simulink model "ad_estimator"  (Simulink 9.3)
settings: Solver=VariableStepAuto  StartTime=0.0  StopTime=10000  MaxStep=0.1  RelTol=1e-3
undefined symbols (not defined in the file or in its folder): a1, a2, b, gam, la
settings Model: Creator=jkord  LastModifiedBy=jkord
settings DataIOCC: SaveFormat=Dataset  SignalLoggingSaveFormat=Dataset  ReturnWorkspaceOutputs=on
settings OptimizationCC: LifeSpan=auto
settings DebuggingCC: UnderspecifiedInitializationDetection=Simplified  MergeDetectMultiDrivingBlocksExec=error  FcnCallInpInsideContextMsg=error  SFUnexpectedBacktrackingDiag=error  SFNoUnconditionalDefaultTransitionDiag=error  SFExecutionAtInitializationDiag=warning  ArithmeticOperatorsInVariantConditions=error
settings HardwareCC: ProdBitPerPointer=64  ProdBitPerSizeT=64  ProdBitPerPtrDiffT=64  ProdLargestAtomicFloat=Float  ProdIntDivRoundTo=Zero  ProdEndianess=LittleEndian  ProdWordSize=64  ProdHWDeviceType=Intel->x86-64 (Windows64)
settings ModelReferenceCC: PropagateSignalLabelsOutOfModel=on
settings SFSimCC: SimUseLocalCustomCode=on
settings RTWCC: RTWUseLocalCustomCode=on
settings CodeAppCC: StateflowObjectComments=off
settings GRTTargetCC: TargetLangStandard=C99 (ISO)  CombineOutputUpdateFcns=on  GRTInterface=off
settings ConfigComp: CovMetricSettings=dwe  CovHtmlReporting=off  CovSaveCumulativeToWorkspaceVar=off  CovSaveSingleToWorkspaceVar=off  CovExternalEMLEnable=on

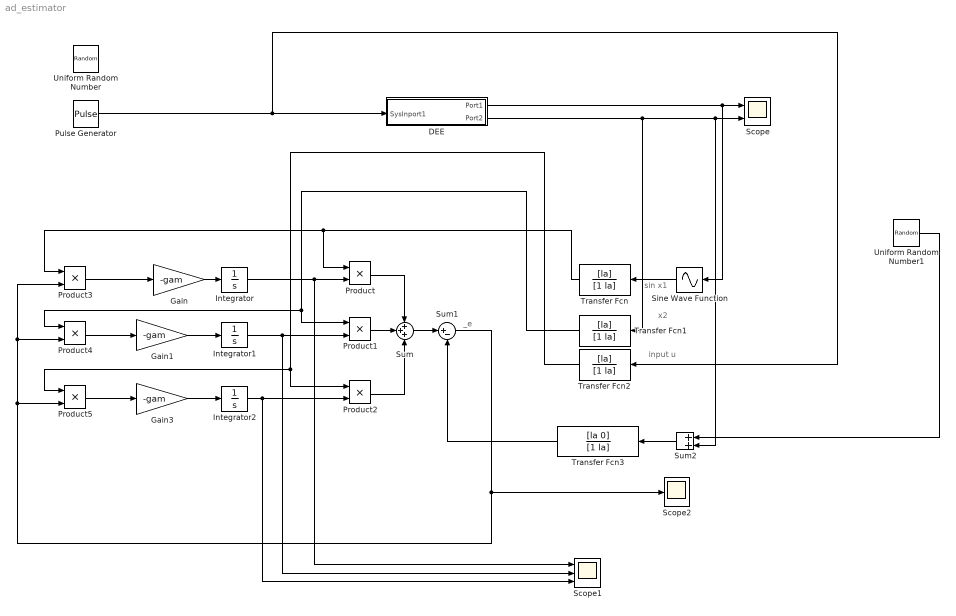
== system ad_estimator ==
  note: _e
  note: input u
  note: x2
  note: sin x1
  DEE : Subsystem  mask(Differential Equation Editor (DEE)){}
      settings: OpenFcn=diffeqed
      mask Display: disp('Differential Equation\n Editor')
  Gain : Gain  Gain=-gam
  Gain1 : Gain  Gain=-gam
  Gain3 : Gain  Gain=-gam
  Integrator : Integrator
  Integrator1 : Integrator
  Integrator2 : Integrator
  Product{,1..5} (6 alike) : Product
  Pulse Generator : DiscretePulseGenerator  PulseType=Time based  Amplitude=0.2  Period=50  PulseWidth=50
  Scope : Scope  NumInputPorts=2
  Scope1 : Scope  NumInputPorts=3
  Scope2 : Scope
  Sine Wave Function : Sin  TimeSource=Use external signal  SampleTime=0
  Sum : Sum  Inputs=+++
  Sum1 : Sum  Inputs=|+-
  Sum2 : Sum
  Transfer Fcn : TransferFcn  Numerator=[la]  Denominator=[1 la]
  Transfer Fcn1 : TransferFcn  Numerator=[la]  Denominator=[1 la]
  Transfer Fcn2 : TransferFcn  Numerator=[la]  Denominator=[1 la]
  Transfer Fcn3 : TransferFcn  Numerator=[la 0]  Denominator=[1 la]
  Uniform Random Number : UniformRandomNumber  SampleTime=0.1
  Uniform Random Number1 : UniformRandomNumber  Minimum=-0.2  Maximum=0.2  SampleTime=0.1
  wires:
  DEE/1(Port1) -> Sine Wave Function/1, Scope/1
  DEE/2(Port2) -> Transfer Fcn1/1, Sum2/2, Scope/2
  Sine Wave Function/1 -> Transfer Fcn/1
  Integrator/1 -> Scope1/1, Product/2
  Integrator1/1 -> Scope1/2, Product1/2
  Integrator2/1 -> Scope1/3, Product2/2
  Product1/1 -> Sum/2
  Product/1 -> Sum/1
  Product2/1 -> Sum/3
  Sum/1 -> Sum1/1
  Transfer Fcn3/1 -> Sum1/2
  Product3/1 -> Gain/1
  Sum1/1 -> Product5/2, Product3/2, Product4/2, Scope2/1
  Product4/1 -> Gain1/1
  Product5/1 -> Gain3/1
  Gain/1 -> Integrator/1
  Gain1/1 -> Integrator1/1
  Gain3/1 -> Integrator2/1
  Transfer Fcn/1 -> Product/1, Product3/1
  Transfer Fcn1/1 -> Product1/1, Product4/1
  Transfer Fcn2/1 -> Product2/1, Product5/1
  Pulse Generator/1 -> DEE/1(SysInport1), Transfer Fcn2/1
  Uniform Random Number1/1 -> Sum2/1
  Sum2/1 -> Transfer Fcn3/1

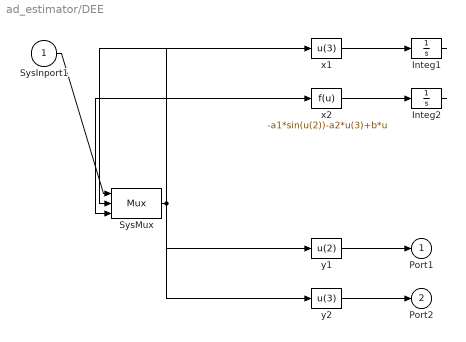
== system ad_estimator/DEE ==
  SysInport1 : Inport
  Integ1 : Integrator
  Integ2 : Integrator
  SysMux : Mux  Inputs=3
  x1 : Fcn  Expr=u(3)
  x2 : Fcn  Expr=-a1*sin(u(2))-a2*u(3)+b*u
  y1 : Fcn  Expr=u(2)
  y2 : Fcn  Expr=u(3)
  Port1 : Outport
  Port2 : Outport  Port=2
  wires:
  SysInport1/1 -> SysMux/1
  SysMux/1 -> x1/1, x2/1, y1/1, y2/1
  x1/1 -> Integ1/1
  Integ1/1 -> SysMux/2
  x2/1 -> Integ2/1
  Integ2/1 -> SysMux/3
  y1/1 -> Port1/1
  y2/1 -> Port2/1
